simulink model "BasicQuadrotorControl"  (R2015a)
settings: Solver=FixedStepDiscrete  StartTime=0.0  StopTime=100000  RelTol=1e-3
model workspace (MAT data in the model file):
  clk_freq = Simulink.Parameter
  clk_freq.Value = 1000000
  clk_freq.DataType = 'uint32'
  cs_to_clk_edge = Simulink.Parameter
  cs_to_clk_edge.Value = 10
  cs_to_clk_edge.DataType = 'uint16'
  DATA_FORMAT = 12552
  init_cmd_ADXL = [11528 11528 11528 12552 12552]
  message_length = Simulink.Parameter
  message_length.Value = 16
  message_length.DataType = 'uint16'
  OUT_X_H = 45824
  OUT_X_L = 45568
  OUT_Y_H = 46336
  OUT_Y_L = 46080
  OUT_Z_H = 46848
  OUT_Z_L = 46592
  POWER_CTRL = 11528
  read_table_ADXL = [45568 45824 46080 46336 46592 46848 32768]
  stall_time = Simulink.Parameter
  stall_time.Value = 4
  stall_time.DataType = 'uint16'
  CTRL_REG1_L3G = 8399
  init_cmd_L3G = 8399
  OUT_X_H_L3G = 43264
  OUT_X_L_L3G = 43008
  OUT_Y_H_L3G = 43776
  OUT_Y_L_L3G = 43520
  OUT_Z_H_L3G = 44288
  OUT_Z_L_L3G = 44032
  read_table_L3G = [43008 43264 43520 43776 44032 44288 36608]
  WHO_AM_I_L3G = 36608
undefined symbols (not defined in the file): read_table
libraries: simulink x20, hdlsllib x2
settings Model: CovSFcnEnable=off  Creator=bsoheili  LastModifiedBy=dlwalter
settings DataIOCC: SaveOutput=off  SaveTime=off
settings OptimizationCC: BlockReduction=off  ConditionallyExecuteInputs=off  InlineParams=on  UseDivisionForNetSlopeComputation=UseDivisionForReciprocalsOfIntegersOnly  UseFloatMulNetSlope=on  InlineInvariantSignals=on  EnhancedBackFolding=on  EfficientFloat2IntCast=on  OptimizeModelRefInitCode=on  LifeSpan=1
settings DebuggingCC: AlgebraicLoopMsg=error  SolverPrmCheckMsg=warning  InheritedTsInSrcMsg=none  StrictBusMsg=ErrorOnBusTreatedAsVector  NonBusSignalsTreatedAsBus=error
settings HardwareCC: ProdHWDeviceType=ASIC/FPGA->ASIC/FPGA  ProdEqTarget=off
settings RTWCC: SystemTargetFile=ert.tlc  TemplateMakefile=ert_default_tmf  Description=Embedded Coder  GenerateReport=on  IncludeHyperlinkInReport=on  LaunchReport=on  GenerateTraceInfo=on  GenerateTraceReport=on  GenerateTraceReportSl=on  GenerateTraceReportSf=on  GenerateTraceReportEml=on  GenerateCodeMetricsReport=on
settings CodeAppCC: IgnoreCustomStorageClasses=off
settings ERTTargetCC: ParMdlRefBuildCompliant=on  CompOptLevelCompliant=on  ConcurrentExecutionCompliant=on  CombineSignalStateStructs=on  SuppressErrorStatus=on  ERTFirstTimeCompliant=on  SupportContinuousTime=off  SupportVariableSizeSignals=off  ModelStepFunctionPrototypeControlCompliant=on  CPPClassGenCompliant=on  ERTCustomFileTemplate=example_file_process.tlc

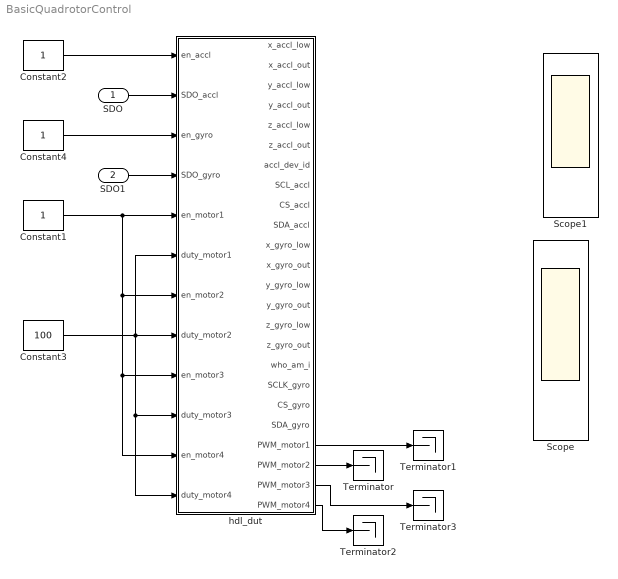
== system BasicQuadrotorControl ==
  SDO : Inport  OutDataTypeStr=boolean
  SDO1 : Inport  Port=2  OutDataTypeStr=boolean
  Constant1 : Constant  OutDataTypeStr=boolean  SampleTime=-1
  Constant2 : Constant  OutDataTypeStr=boolean  SampleTime=-1
  Constant3 : Constant  Value=100  OutDataTypeStr=uint8  SampleTime=-1
  Constant4 : Constant  OutDataTypeStr=boolean  SampleTime=-1
  Scope : Scope  NumInputPorts=4
      settings: TickLabels=on  TimeRange=2000  YMin=-5~-5~-5~-5  YMax=5~5~5~5
  Scope1 : Scope  NumInputPorts=4
      settings: TickLabels=on  TimeRange=2000  YMin=-5~-5~-5~-5  YMax=5~5~5~5  SaveName=ScopeData2
  Terminator{,1..3} (4 alike) : Terminator
  hdl_dut : Subsystem  TreatAsAtomicUnit=on
  wires:
  SDO/1 -> hdl_dut/2(SDO_accl)
  Constant3/1 -> hdl_dut/6(duty_motor1), hdl_dut/10(duty_motor3), hdl_dut/12(duty_motor4), hdl_dut/8(duty_motor2)
  Constant1/1 -> hdl_dut/5(en_motor1), hdl_dut/9(en_motor3), hdl_dut/11(en_motor4), hdl_dut/7(en_motor2)
  Constant2/1 -> hdl_dut/1(en_accl)
  Constant4/1 -> hdl_dut/3(en_gyro)
  SDO1/1 -> hdl_dut/4(SDO_gyro)
  hdl_dut/21(PWM_motor1) -> Terminator1/1
  hdl_dut/22(PWM_motor2) -> Terminator/1
  hdl_dut/23(PWM_motor3) -> Terminator3/1
  hdl_dut/24(PWM_motor4) -> Terminator2/1

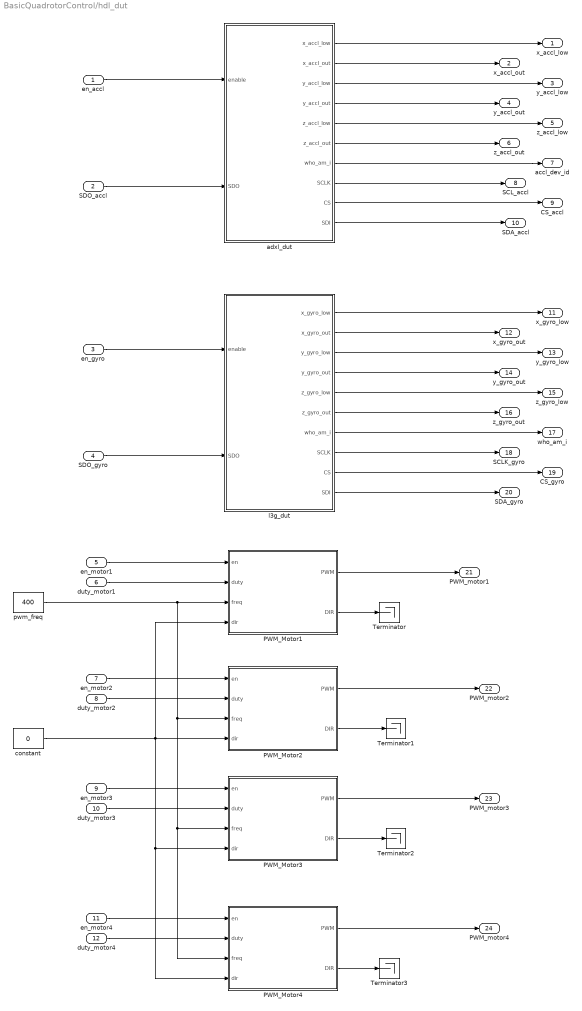
== system BasicQuadrotorControl/hdl_dut ==
  en_accl : Inport
  SDO_accl : Inport  Port=2
  en_gyro : Inport  Port=3
  SDO_gyro : Inport  Port=4
  en_motor1 : Inport  Port=5
  duty_motor1 : Inport  Port=6
  en_motor2 : Inport  Port=7
  duty_motor2 : Inport  Port=8
  en_motor3 : Inport  Port=9
  duty_motor3 : Inport  Port=10
  en_motor4 : Inport  Port=11
  duty_motor4 : Inport  Port=12
  PWM_Motor1 : Subsystem
  PWM_Motor2 : Subsystem
  PWM_Motor3 : Subsystem
  PWM_Motor4 : Subsystem
  Terminator{,1..3} (4 alike) : Terminator
  adxl_dut : Subsystem  TreatAsAtomicUnit=on  MinMaxOverflowLogging=MinMaxAndOverflow
  constant : Constant  Value=0  OutDataTypeStr=boolean  SampleTime=-1
  l3g_dut : Subsystem  TreatAsAtomicUnit=on  MinMaxOverflowLogging=MinMaxAndOverflow
  pwm_freq : Constant  Value=400  OutDataTypeStr=uint32  SampleTime=-1
  x_accl_low : Outport
  x_accl_out : Outport  Port=2
  y_accl_low : Outport  Port=3
  y_accl_out : Outport  Port=4
  z_accl_low : Outport  Port=5
  z_accl_out : Outport  Port=6
  accl_dev_id : Outport  Port=7
  SCL_accl : Outport  Port=8
  CS_accl : Outport  Port=9
  SDA_accl : Outport  Port=10
  x_gyro_low : Outport  Port=11
  x_gyro_out : Outport  Port=12
  y_gyro_low : Outport  Port=13
  y_gyro_out : Outport  Port=14
  z_gyro_low : Outport  Port=15
  z_gyro_out : Outport  Port=16
  who_am_i : Outport  Port=17
  SCLK_gyro : Outport  Port=18
  CS_gyro : Outport  Port=19
  SDA_gyro : Outport  Port=20
  PWM_motor1 : Outport  Port=21  OutDataTypeStr=boolean
  PWM_motor2 : Outport  Port=22  OutDataTypeStr=boolean
  PWM_motor3 : Outport  Port=23  OutDataTypeStr=boolean
  PWM_motor4 : Outport  Port=24  OutDataTypeStr=boolean
  wires:
  en_accl/1 -> adxl_dut/1(enable)
  SDO_accl/1 -> adxl_dut/2(SDO)
  adxl_dut/3(y_accl_low) -> y_accl_low/1
  adxl_dut/1(x_accl_low) -> x_accl_low/1
  pwm_freq/1 -> PWM_Motor4/3(freq), PWM_Motor3/3(freq), PWM_Motor2/3(freq), PWM_Motor1/3(freq)
  en_motor1/1 -> PWM_Motor1/1(en)
  duty_motor1/1 -> PWM_Motor1/2(duty)
  en_motor2/1 -> PWM_Motor2/1(en)
  duty_motor2/1 -> PWM_Motor2/2(duty)
  constant/1 -> PWM_Motor2/4(dir), PWM_Motor3/4(dir), PWM_Motor4/4(dir), PWM_Motor1/4(dir)
  PWM_Motor1/1(PWM) -> PWM_motor1/1
  PWM_Motor2/1(PWM) -> PWM_motor2/1
  PWM_Motor1/2(DIR) -> Terminator/1
  PWM_Motor2/2(DIR) -> Terminator1/1
  PWM_Motor3/2(DIR) -> Terminator2/1
  PWM_Motor4/2(DIR) -> Terminator3/1
  PWM_Motor3/1(PWM) -> PWM_motor3/1
  PWM_Motor4/1(PWM) -> PWM_motor4/1
  en_motor3/1 -> PWM_Motor3/1(en)
  duty_motor3/1 -> PWM_Motor3/2(duty)
  en_motor4/1 -> PWM_Motor4/1(en)
  duty_motor4/1 -> PWM_Motor4/2(duty)
  adxl_dut/10(SDI) -> SDA_accl/1
  adxl_dut/8(SCLK) -> SCL_accl/1
  adxl_dut/2(x_accl_out) -> x_accl_out/1
  adxl_dut/4(y_accl_out) -> y_accl_out/1
  adxl_dut/5(z_accl_low) -> z_accl_low/1
  adxl_dut/6(z_accl_out) -> z_accl_out/1
  adxl_dut/7(who_am_i) -> accl_dev_id/1
  en_gyro/1 -> l3g_dut/1(enable)
  SDO_gyro/1 -> l3g_dut/2(SDO)
  l3g_dut/10(SDI) -> SDA_gyro/1
  l3g_dut/8(SCLK) -> SCLK_gyro/1
  l3g_dut/1(x_gyro_low) -> x_gyro_low/1
  l3g_dut/2(x_gyro_out) -> x_gyro_out/1
  l3g_dut/3(y_gyro_low) -> y_gyro_low/1
  l3g_dut/4(y_gyro_out) -> y_gyro_out/1
  l3g_dut/5(z_gyro_low) -> z_gyro_low/1
  l3g_dut/6(z_gyro_out) -> z_gyro_out/1
  l3g_dut/7(who_am_i) -> who_am_i/1
  adxl_dut/9(CS) -> CS_accl/1
  l3g_dut/9(CS) -> CS_gyro/1

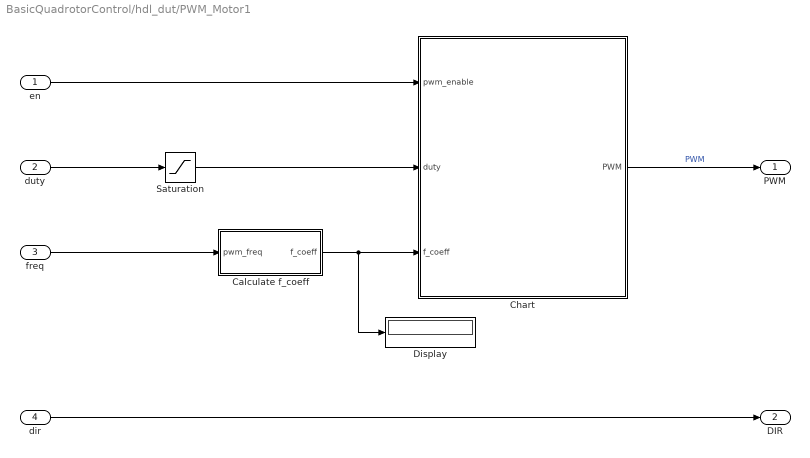
== system BasicQuadrotorControl/hdl_dut/PWM_Motor1 ==
  en : Inport  OutDataTypeStr=boolean  PortDimensions=1  SampleTime=[1,0]
  duty : Inport  Port=2  OutDataTypeStr=uint8  PortDimensions=1  SampleTime=[1,0]
  freq : Inport  Port=3  OutDataTypeStr=uint32  PortDimensions=1  SampleTime=[1,0]
  dir : Inport  Port=4  OutDataTypeStr=boolean  PortDimensions=1  SampleTime=[1,0]
  Calculate f_coeff : Subsystem  TreatAsAtomicUnit=on
  Chart : Stateflow chart  TreatAsAtomicUnit=on
  Display : Display
  Saturation : Saturate  UpperLimit=255  LowerLimit=0  OutDataTypeStr=fixdt(0,8,0)
  PWM : Outport  OutDataTypeStr=boolean  PortDimensions=1  SampleTime=[1,0]
  DIR : Outport  Port=2  PortDimensions=1  SampleTime=[1,0]
  wires:
  dir/1 -> DIR/1
  en/1 -> Chart/1(pwm_enable)
  duty/1 -> Saturation/1
  Saturation/1 -> Chart/2(duty)
  Chart/1(PWM) -> PWM/1  "PWM"
  freq/1 -> Calculate f_coeff/1(pwm_freq)
  Calculate f_coeff/1(f_coeff) -> Chart/3(f_coeff), Display/1

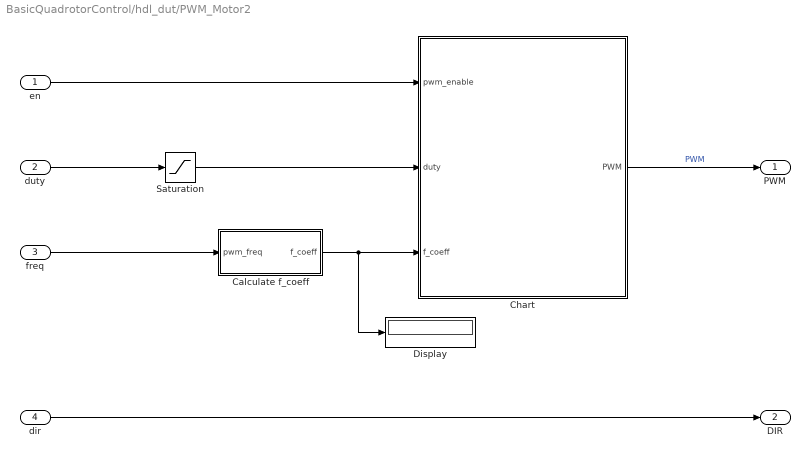
== system BasicQuadrotorControl/hdl_dut/PWM_Motor2 ==
  en : Inport  OutDataTypeStr=boolean  PortDimensions=1  SampleTime=[1,0]
  duty : Inport  Port=2  OutDataTypeStr=uint8  PortDimensions=1  SampleTime=[1,0]
  freq : Inport  Port=3  OutDataTypeStr=uint32  PortDimensions=1  SampleTime=[1,0]
  dir : Inport  Port=4  OutDataTypeStr=boolean  PortDimensions=1  SampleTime=[1,0]
  Calculate f_coeff : Subsystem  TreatAsAtomicUnit=on
  Chart : Stateflow chart  TreatAsAtomicUnit=on
  Display : Display
  Saturation : Saturate  UpperLimit=255  LowerLimit=0  OutDataTypeStr=fixdt(0,8,0)
  PWM : Outport  OutDataTypeStr=boolean  PortDimensions=1  SampleTime=[1,0]
  DIR : Outport  Port=2  PortDimensions=1  SampleTime=[1,0]
  wires:
  Calculate f_coeff/1(f_coeff) -> Display/1, Chart/3(f_coeff)
  freq/1 -> Calculate f_coeff/1(pwm_freq)
  Chart/1(PWM) -> PWM/1  "PWM"
  Saturation/1 -> Chart/2(duty)
  duty/1 -> Saturation/1
  en/1 -> Chart/1(pwm_enable)
  dir/1 -> DIR/1

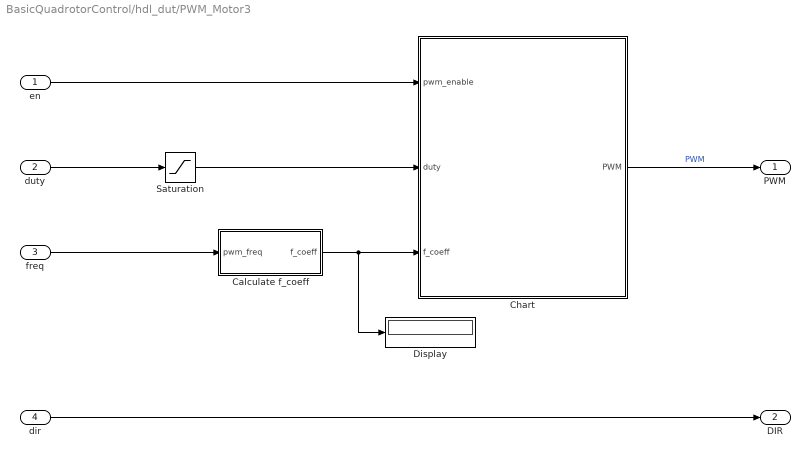
== system BasicQuadrotorControl/hdl_dut/PWM_Motor3 ==
  en : Inport  OutDataTypeStr=boolean  PortDimensions=1  SampleTime=[1,0]
  duty : Inport  Port=2  OutDataTypeStr=uint8  PortDimensions=1  SampleTime=[1,0]
  freq : Inport  Port=3  OutDataTypeStr=uint32  PortDimensions=1  SampleTime=[1,0]
  dir : Inport  Port=4  OutDataTypeStr=boolean  PortDimensions=1  SampleTime=[1,0]
  Calculate f_coeff : Subsystem  TreatAsAtomicUnit=on
  Chart : Stateflow chart  TreatAsAtomicUnit=on
  Display : Display
  Saturation : Saturate  UpperLimit=255  LowerLimit=0  OutDataTypeStr=fixdt(0,8,0)
  PWM : Outport  OutDataTypeStr=boolean  PortDimensions=1  SampleTime=[1,0]
  DIR : Outport  Port=2  PortDimensions=1  SampleTime=[1,0]
  wires:
  dir/1 -> DIR/1
  en/1 -> Chart/1(pwm_enable)
  duty/1 -> Saturation/1
  Saturation/1 -> Chart/2(duty)
  Chart/1(PWM) -> PWM/1  "PWM"
  freq/1 -> Calculate f_coeff/1(pwm_freq)
  Calculate f_coeff/1(f_coeff) -> Chart/3(f_coeff), Display/1

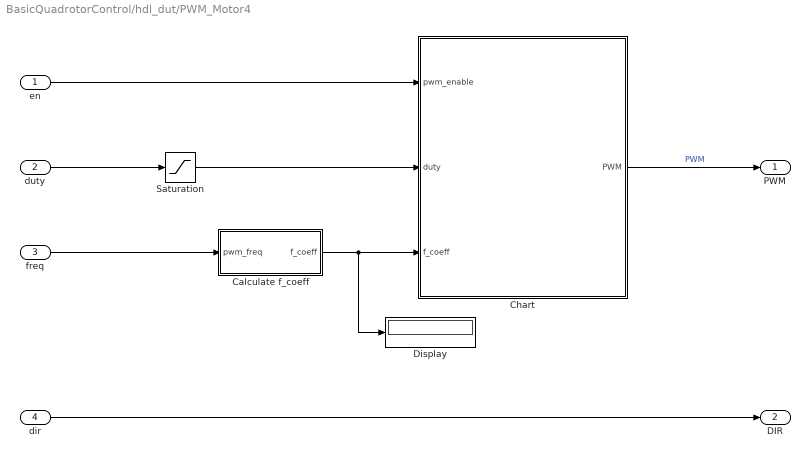
== system BasicQuadrotorControl/hdl_dut/PWM_Motor4 ==
  en : Inport  OutDataTypeStr=boolean  PortDimensions=1  SampleTime=[1,0]
  duty : Inport  Port=2  OutDataTypeStr=uint8  PortDimensions=1  SampleTime=[1,0]
  freq : Inport  Port=3  OutDataTypeStr=uint32  PortDimensions=1  SampleTime=[1,0]
  dir : Inport  Port=4  OutDataTypeStr=boolean  PortDimensions=1  SampleTime=[1,0]
  Calculate f_coeff : Subsystem  TreatAsAtomicUnit=on
  Chart : Stateflow chart  TreatAsAtomicUnit=on
  Display : Display
  Saturation : Saturate  UpperLimit=255  LowerLimit=0  OutDataTypeStr=fixdt(0,8,0)
  PWM : Outport  OutDataTypeStr=boolean  PortDimensions=1  SampleTime=[1,0]
  DIR : Outport  Port=2  PortDimensions=1  SampleTime=[1,0]
  wires:
  Calculate f_coeff/1(f_coeff) -> Display/1, Chart/3(f_coeff)
  freq/1 -> Calculate f_coeff/1(pwm_freq)
  Chart/1(PWM) -> PWM/1  "PWM"
  Saturation/1 -> Chart/2(duty)
  duty/1 -> Saturation/1
  en/1 -> Chart/1(pwm_enable)
  dir/1 -> DIR/1

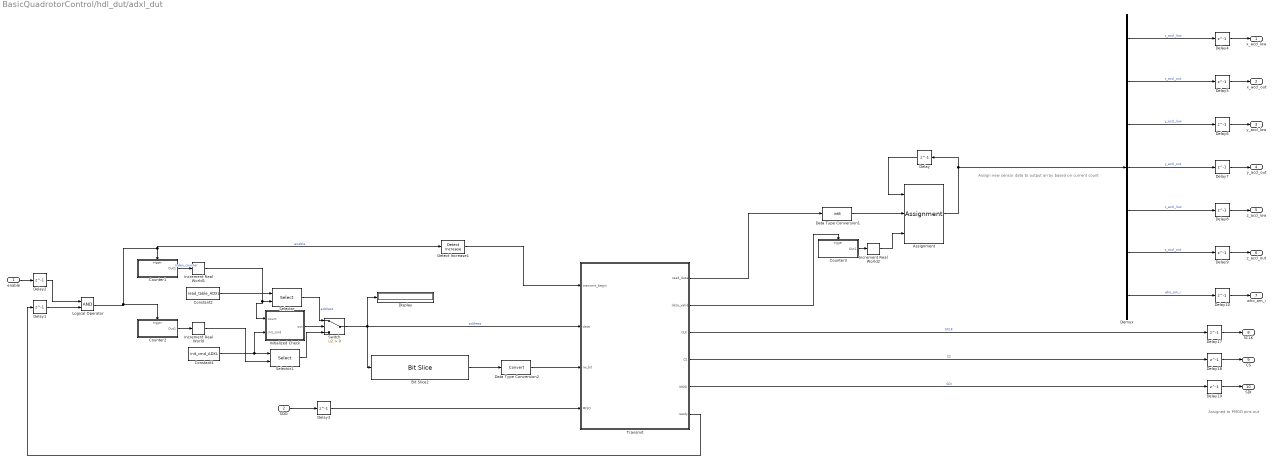
== system BasicQuadrotorControl/hdl_dut/adxl_dut ==
  note: Assign new sensor data to output array based on current count
  note: Assigned to PMOD pins out
  enable : Inport
  SDO : Inport  Port=2
  Assignment : Assignment  DiagnosticForDimensions=Warning  IndexOptions=Index vector (port)  OutputSizes=size(read_table,2)
  Bit Slice2 : hdlsllib/HDL Operations/Bit Slice  lidx=message_length-1  ridx=message_length-1
  Constant1 : Constant  Value=init_cmd_ADXL  OutDataTypeStr=uint16  SampleTime=1
  Constant2 : Constant  Value=read_table_ADXL  OutDataTypeStr=uint16  SampleTime=1
  Counter1 : Subsystem  TreatAsAtomicUnit=on
  Counter2 : Subsystem  TreatAsAtomicUnit=on
  Counter3 : Subsystem  TreatAsAtomicUnit=on
  Data Type Conversion1 : DataTypeConversion  OutDataTypeStr=int8  ConvertRealWorld=Stored Integer (SI)
  Data Type Conversion2 : DataTypeConversion
  Delay : Delay  DelayLength=1  InitialCondition=zeros(1,size(read_table_ADXL,2))  SampleTime=1
  Delay1 : Delay  DelayLength=1  InitialCondition=1
  Delay{4..10,17..19} (10 alike) : Delay  DelayLength=1  InitialCondition=0
  Delay2 : Delay  DelayLength=1  InitialCondition=1
  Delay3 : Delay  DelayLength=1  InitialCondition=1
  Demux : Demux  Outputs=7
  Detect Increase1 : simulink/Logic and Bit Operations/Detect Increase  vinit=0  InputProcessing=Inherited  OutDataTypeStr=boolean
  Display : Display
      settings: Format=binary (Stored Integer)
  Increment Real World : simulink/Additional Math & Discrete/Additional Math: Increment - Decrement/Increment Real World
  Increment Real World1 : simulink/Additional Math & Discrete/Additional Math: Increment - Decrement/Increment Real World
  Increment Real World2 : simulink/Additional Math & Discrete/Additional Math: Increment - Decrement/Increment Real World
  Initialized Check : MATLAB Function  TreatAsAtomicUnit=on
  Logical Operator : Logic  AllPortsSameDT=off  OutDataTypeStr=boolean
  Selector : Selector  InputPortWidth=size(read_table_ADXL,2)  IndexOptions=Index vector (port)  Indices=[1 3]
  Selector1 : Selector  InputPortWidth=size(init_cmd_ADXL,2)  IndexOptions=Index vector (port)  Indices=[1 3]
  Switch : Switch  Criteria=u2 > Threshold
  Transmit : Stateflow chart  TreatAsAtomicUnit=on
  x_accl_low : Outport
  x_accl_out : Outport  Port=2
  y_accl_low : Outport  Port=3
  y_accl_out : Outport  Port=4
  z_accl_low : Outport  Port=5
  z_accl_out : Outport  Port=6
  who_am_i : Outport  Port=7
  SCLK : Outport  Port=8
  CS : Outport  Port=9
  SDI : Outport  Port=10
  wires:
  Transmit/3(CLK) -> Delay17/1  "SCLK"
  Transmit/4(CS) -> Delay18/1  "CS"
  Transmit/5(MOSI) -> Delay19/1  "SDI"
  Assignment/1 -> Delay/1, Demux/1
  enable/1 -> Delay2/1
  Constant2/1 -> Selector/1
  Transmit/6(ready) -> Delay1/1
  SDO/1 -> Delay3/1
  Delay1/1 -> Logical Operator/2
  Counter1/1(Out1) -> Increment Real World1/1  "index_counter"
  Delay/1 -> Assignment/1
  Delay2/1 -> Logical Operator/1
  Delay4/1 -> x_accl_low/1
  Delay5/1 -> x_accl_out/1
  Delay6/1 -> y_accl_low/1
  Delay7/1 -> y_accl_out/1
  Delay8/1 -> z_accl_low/1
  Delay9/1 -> z_accl_out/1
  Delay10/1 -> who_am_i/1
  Delay17/1 -> SCLK/1
  Delay18/1 -> CS/1
  Delay19/1 -> SDI/1
  Detect Increase1/1 -> Transmit/1(transmit_begin)
  Logical Operator/1 -> Counter2/Trigger, Counter1/Trigger, Detect Increase1/1  "enable"
  Delay3/1 -> Transmit/4(MISO)
  Data Type Conversion2/1 -> Transmit/3(rw_bit)
  Switch/1 -> Display/1, Transmit/2(data), Bit Slice2/1  "address"
  Bit Slice2/1 -> Data Type Conversion2/1
  Demux/1 -> Delay4/1  "x_accl_low"
  Demux/2 -> Delay5/1  "x_accl_out"
  Demux/3 -> Delay6/1  "y_accl_low"
  Demux/4 -> Delay7/1  "y_accl_out"
  Demux/5 -> Delay8/1  "z_accl_low"
  Demux/6 -> Delay9/1  "z_accl_out"
  Demux/7 -> Delay10/1  "who_am_i"
  Transmit/1(read_data) -> Data Type Conversion1/1
  Data Type Conversion1/1 -> Assignment/2
  Counter3/1(Out1) -> Increment Real World2/1
  Transmit/2(data_valid) -> Counter3/Trigger
  Selector/1 -> Switch/1  "address"
  Selector1/1 -> Switch/3
  Constant1/1 -> Selector1/1, Initialized Check/2(init_cmd)
  Counter2/1(Out1) -> Increment Real World/1
  Increment Real World/1 -> Selector1/2
  Increment Real World1/1 -> Initialized Check/1(count), Selector/2
  Increment Real World2/1 -> Assignment/3
  Initialized Check/1(out) -> Switch/2

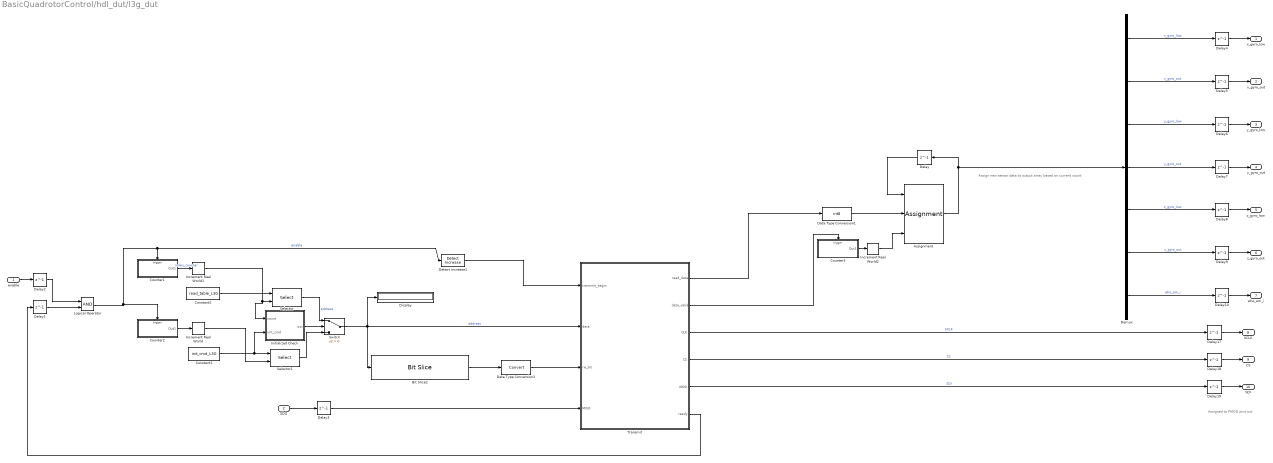
== system BasicQuadrotorControl/hdl_dut/l3g_dut ==
  note: Assign new sensor data to output array based on current count
  note: Assigned to PMOD pins out
  enable : Inport
  SDO : Inport  Port=2
  Assignment : Assignment  DiagnosticForDimensions=Warning  IndexOptions=Index vector (port)  OutputSizes=size(read_table,2)
  Bit Slice2 : hdlsllib/HDL Operations/Bit Slice  lidx=message_length-1  ridx=message_length-1
  Constant1 : Constant  Value=init_cmd_L3G  OutDataTypeStr=uint16  SampleTime=1
  Constant2 : Constant  Value=read_table_L3G  OutDataTypeStr=uint16  SampleTime=1
  Counter1 : Subsystem  TreatAsAtomicUnit=on
  Counter2 : Subsystem  TreatAsAtomicUnit=on
  Counter3 : Subsystem  TreatAsAtomicUnit=on
  Data Type Conversion1 : DataTypeConversion  OutDataTypeStr=int8  ConvertRealWorld=Stored Integer (SI)
  Data Type Conversion2 : DataTypeConversion
  Delay : Delay  DelayLength=1  InitialCondition=zeros(1,size(read_table_L3G,2))  SampleTime=1
  Delay1 : Delay  DelayLength=1  InitialCondition=1
  Delay{4..10,17..19} (10 alike) : Delay  DelayLength=1  InitialCondition=0
  Delay2 : Delay  DelayLength=1  InitialCondition=1
  Delay3 : Delay  DelayLength=1  InitialCondition=1
  Demux : Demux  Outputs=7
  Detect Increase1 : simulink/Logic and Bit Operations/Detect Increase  vinit=0  InputProcessing=Inherited  OutDataTypeStr=boolean
  Display : Display
      settings: Format=binary (Stored Integer)
  Increment Real World : simulink/Additional Math & Discrete/Additional Math: Increment - Decrement/Increment Real World
  Increment Real World1 : simulink/Additional Math & Discrete/Additional Math: Increment - Decrement/Increment Real World
  Increment Real World2 : simulink/Additional Math & Discrete/Additional Math: Increment - Decrement/Increment Real World
  Initialized Check : MATLAB Function  TreatAsAtomicUnit=on
  Logical Operator : Logic  AllPortsSameDT=off  OutDataTypeStr=boolean
  Selector : Selector  InputPortWidth=size(read_table_L3G,2)  IndexOptions=Index vector (port)  Indices=[1 3]
  Selector1 : Selector  InputPortWidth=size(init_cmd_L3G,2)  IndexOptions=Index vector (port)  Indices=[1 3]
  Switch : Switch  Criteria=u2 > Threshold
  Transmit : Stateflow chart  TreatAsAtomicUnit=on
  x_gyro_low : Outport
  x_gyro_out : Outport  Port=2
  y_gyro_low : Outport  Port=3
  y_gyro_out : Outport  Port=4
  z_gyro_low : Outport  Port=5
  z_gyro_out : Outport  Port=6
  who_am_i : Outport  Port=7
  SCLK : Outport  Port=8
  CS : Outport  Port=9
  SDI : Outport  Port=10
  wires:
  Transmit/3(CLK) -> Delay17/1  "SCLK"
  Transmit/4(CS) -> Delay18/1  "CS"
  Transmit/5(MOSI) -> Delay19/1  "SDI"
  Assignment/1 -> Delay/1, Demux/1
  enable/1 -> Delay2/1
  Constant2/1 -> Selector/1
  Transmit/6(ready) -> Delay1/1
  SDO/1 -> Delay3/1
  Delay1/1 -> Logical Operator/2
  Counter1/1(Out1) -> Increment Real World1/1  "index_counter"
  Delay/1 -> Assignment/1
  Delay2/1 -> Logical Operator/1
  Delay4/1 -> x_gyro_low/1
  Delay5/1 -> x_gyro_out/1
  Delay6/1 -> y_gyro_low/1
  Delay7/1 -> y_gyro_out/1
  Delay8/1 -> z_gyro_low/1
  Delay9/1 -> z_gyro_out/1
  Delay10/1 -> who_am_i/1
  Delay17/1 -> SCLK/1
  Delay18/1 -> CS/1
  Delay19/1 -> SDI/1
  Detect Increase1/1 -> Transmit/1(transmit_begin)
  Logical Operator/1 -> Counter2/Trigger, Counter1/Trigger, Detect Increase1/1  "enable"
  Delay3/1 -> Transmit/4(MISO)
  Data Type Conversion2/1 -> Transmit/3(rw_bit)
  Switch/1 -> Display/1, Transmit/2(data), Bit Slice2/1  "address"
  Bit Slice2/1 -> Data Type Conversion2/1
  Demux/1 -> Delay4/1  "x_gyro_low"
  Demux/2 -> Delay5/1  "x_gyro_out"
  Demux/3 -> Delay6/1  "y_gyro_low"
  Demux/4 -> Delay7/1  "y_gyro_out"
  Demux/5 -> Delay8/1  "z_gyro_low"
  Demux/6 -> Delay9/1  "z_gyro_out"
  Demux/7 -> Delay10/1  "who_am_i"
  Transmit/1(read_data) -> Data Type Conversion1/1
  Data Type Conversion1/1 -> Assignment/2
  Counter3/1(Out1) -> Increment Real World2/1
  Transmit/2(data_valid) -> Counter3/Trigger
  Selector/1 -> Switch/1  "address"
  Selector1/1 -> Switch/3
  Constant1/1 -> Selector1/1, Initialized Check/2(init_cmd)
  Counter2/1(Out1) -> Increment Real World/1
  Increment Real World/1 -> Selector1/2
  Increment Real World1/1 -> Initialized Check/1(count), Selector/2
  Increment Real World2/1 -> Assignment/3
  Initialized Check/1(out) -> Switch/2

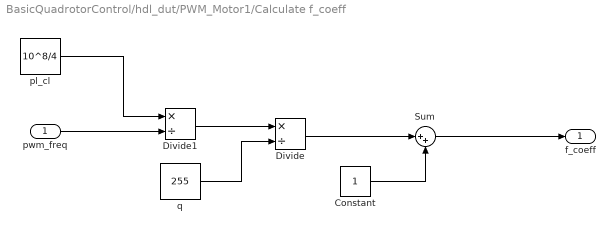
== system BasicQuadrotorControl/hdl_dut/PWM_Motor1/Calculate f_coeff ==
  pwm_freq : Inport
  Constant : Constant  OutDataTypeStr=uint32
  Divide : Product  Inputs=*/  SaturateOnIntegerOverflow=on  RndMeth=Zero
  Divide1 : Product  Inputs=*/  SaturateOnIntegerOverflow=on  RndMeth=Zero
  Sum : Sum  Inputs=|++  AccumDataTypeStr=uint32  RndMeth=Zero
  pl_cl : Constant  Value=10^8/4  OutDataTypeStr=uint32
  q : Constant  Value=255  OutDataTypeStr=Inherit: Inherit via back propagation
  f_coeff : Outport  OutDataTypeStr=uint32
  wires:
  Constant/1 -> Sum/2
  Sum/1 -> f_coeff/1
  Divide/1 -> Sum/1
  pl_cl/1 -> Divide1/1
  pwm_freq/1 -> Divide1/2
  Divide1/1 -> Divide/1
  q/1 -> Divide/2

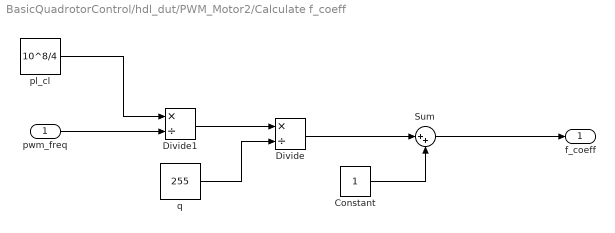
== system BasicQuadrotorControl/hdl_dut/PWM_Motor2/Calculate f_coeff ==
  pwm_freq : Inport
  Constant : Constant  OutDataTypeStr=uint32
  Divide : Product  Inputs=*/  SaturateOnIntegerOverflow=on  RndMeth=Zero
  Divide1 : Product  Inputs=*/  SaturateOnIntegerOverflow=on  RndMeth=Zero
  Sum : Sum  Inputs=|++  AccumDataTypeStr=uint32  RndMeth=Zero
  pl_cl : Constant  Value=10^8/4  OutDataTypeStr=uint32
  q : Constant  Value=255  OutDataTypeStr=Inherit: Inherit via back propagation
  f_coeff : Outport  OutDataTypeStr=uint32
  wires:
  q/1 -> Divide/2
  Divide1/1 -> Divide/1
  pwm_freq/1 -> Divide1/2
  pl_cl/1 -> Divide1/1
  Divide/1 -> Sum/1
  Sum/1 -> f_coeff/1
  Constant/1 -> Sum/2

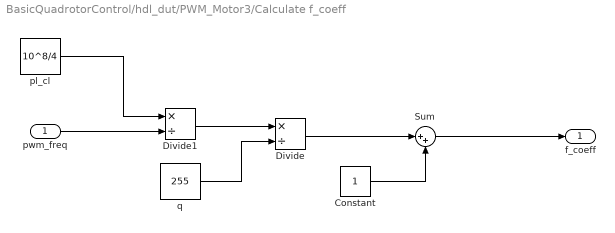
== system BasicQuadrotorControl/hdl_dut/PWM_Motor3/Calculate f_coeff ==
  pwm_freq : Inport
  Constant : Constant  OutDataTypeStr=uint32
  Divide : Product  Inputs=*/  SaturateOnIntegerOverflow=on  RndMeth=Zero
  Divide1 : Product  Inputs=*/  SaturateOnIntegerOverflow=on  RndMeth=Zero
  Sum : Sum  Inputs=|++  AccumDataTypeStr=uint32  RndMeth=Zero
  pl_cl : Constant  Value=10^8/4  OutDataTypeStr=uint32
  q : Constant  Value=255  OutDataTypeStr=Inherit: Inherit via back propagation
  f_coeff : Outport  OutDataTypeStr=uint32
  wires:
  Constant/1 -> Sum/2
  Sum/1 -> f_coeff/1
  Divide/1 -> Sum/1
  pl_cl/1 -> Divide1/1
  pwm_freq/1 -> Divide1/2
  Divide1/1 -> Divide/1
  q/1 -> Divide/2

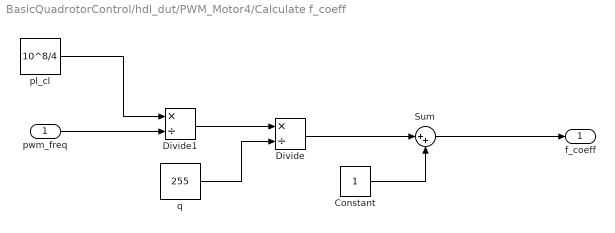
== system BasicQuadrotorControl/hdl_dut/PWM_Motor4/Calculate f_coeff ==
  pwm_freq : Inport
  Constant : Constant  OutDataTypeStr=uint32
  Divide : Product  Inputs=*/  SaturateOnIntegerOverflow=on  RndMeth=Zero
  Divide1 : Product  Inputs=*/  SaturateOnIntegerOverflow=on  RndMeth=Zero
  Sum : Sum  Inputs=|++  AccumDataTypeStr=uint32  RndMeth=Zero
  pl_cl : Constant  Value=10^8/4  OutDataTypeStr=uint32
  q : Constant  Value=255  OutDataTypeStr=Inherit: Inherit via back propagation
  f_coeff : Outport  OutDataTypeStr=uint32
  wires:
  q/1 -> Divide/2
  Divide1/1 -> Divide/1
  pwm_freq/1 -> Divide1/2
  pl_cl/1 -> Divide1/1
  Divide/1 -> Sum/1
  Sum/1 -> f_coeff/1
  Constant/1 -> Sum/2

== system BasicQuadrotorControl/hdl_dut/adxl_dut/Counter1 ==
  Trigger : TriggerPort  PortDimensions=1
  Delay : Delay  DelayLength=1  InitialCondition=1
  Increment Real World : simulink/Additional Math & Discrete/Additional Math: Increment - Decrement/Increment Real World
  Wrap To Zero : simulink/Discontinuities/Wrap To Zero  DisableCoverage=on  Threshold=size(read_table_ADXL,2)-1
  Out1 : Outport  OutDataTypeStr=int16  InitialOutput=0
  wires:
  Delay/1 -> Wrap To Zero/1
  Increment Real World/1 -> Delay/1
  Wrap To Zero/1 -> Out1/1, Increment Real World/1

== system BasicQuadrotorControl/hdl_dut/adxl_dut/Counter2 ==
  Trigger : TriggerPort  PortDimensions=1
  Delay : Delay  DelayLength=1  InitialCondition=1
  Increment Real World : simulink/Additional Math & Discrete/Additional Math: Increment - Decrement/Increment Real World
  Wrap To Zero : simulink/Discontinuities/Wrap To Zero  DisableCoverage=on  Threshold=size(init_cmd_ADXL,2)-1
  Out1 : Outport  OutDataTypeStr=int16  InitialOutput=0
  wires:
  Wrap To Zero/1 -> Increment Real World/1, Out1/1
  Increment Real World/1 -> Delay/1
  Delay/1 -> Wrap To Zero/1

== system BasicQuadrotorControl/hdl_dut/adxl_dut/Counter3 ==
  Trigger : TriggerPort  PortDimensions=1
  Delay : Delay  DelayLength=1  InitialCondition=0
  Increment Real World : simulink/Additional Math & Discrete/Additional Math: Increment - Decrement/Increment Real World
  Wrap To Zero : simulink/Discontinuities/Wrap To Zero  DisableCoverage=on  Threshold=size(read_table_ADXL,2)-1
  Out1 : Outport  OutDataTypeStr=int16  InitialOutput=0
  wires:
  Wrap To Zero/1 -> Increment Real World/1, Out1/1
  Increment Real World/1 -> Delay/1
  Delay/1 -> Wrap To Zero/1

== system BasicQuadrotorControl/hdl_dut/l3g_dut/Counter1 ==
  Trigger : TriggerPort  PortDimensions=1
  Delay : Delay  DelayLength=1  InitialCondition=1
  Increment Real World : simulink/Additional Math & Discrete/Additional Math: Increment - Decrement/Increment Real World
  Wrap To Zero : simulink/Discontinuities/Wrap To Zero  DisableCoverage=on  Threshold=size(read_table_L3G,2)-1
  Out1 : Outport  OutDataTypeStr=int16  InitialOutput=0
  wires:
  Delay/1 -> Wrap To Zero/1
  Increment Real World/1 -> Delay/1
  Wrap To Zero/1 -> Out1/1, Increment Real World/1

== system BasicQuadrotorControl/hdl_dut/l3g_dut/Counter2 ==
  Trigger : TriggerPort  PortDimensions=1
  Delay : Delay  DelayLength=1  InitialCondition=1
  Increment Real World : simulink/Additional Math & Discrete/Additional Math: Increment - Decrement/Increment Real World
  Wrap To Zero : simulink/Discontinuities/Wrap To Zero  DisableCoverage=on  Threshold=size(init_cmd_L3G,2)-1
  Out1 : Outport  OutDataTypeStr=int16  InitialOutput=0
  wires:
  Wrap To Zero/1 -> Increment Real World/1, Out1/1
  Increment Real World/1 -> Delay/1
  Delay/1 -> Wrap To Zero/1

== system BasicQuadrotorControl/hdl_dut/l3g_dut/Counter3 ==
  Trigger : TriggerPort  PortDimensions=1
  Delay : Delay  DelayLength=1  InitialCondition=0
  Increment Real World : simulink/Additional Math & Discrete/Additional Math: Increment - Decrement/Increment Real World
  Wrap To Zero : simulink/Discontinuities/Wrap To Zero  DisableCoverage=on  Threshold=size(read_table_L3G,2)-1
  Out1 : Outport  OutDataTypeStr=int16  InitialOutput=0
  wires:
  Wrap To Zero/1 -> Increment Real World/1, Out1/1
  Increment Real World/1 -> Delay/1
  Delay/1 -> Wrap To Zero/1

== stateflow chart BasicQuadrotorControl/hdl_dut/adxl_dut/Transmit ==
  settings: executeAtInitialization=1
  state IDLE
  state BEGIN
  state CHIPSELECT
  state WRITE
    state CLOCK_BEGIN
    state CLOCK_HIGH
    state CLOCK_LOW
    state CLOCK_END
    (default) -> CLOCK_BEGIN
    CLOCK_BEGIN -> CLOCK_LOW : {CLK = false;
        | bit_count = 0;
        | MOSI = sdi_gen(data,1);}
    CLOCK_LOW -> CLOCK_HIGH [order 1] : [count == clk_wait]
        | {CLK = 1; count = 0;bit_count ++;}
    CLOCK_HIGH -> CLOCK_HIGH [order 3] : {count++;}
    CLOCK_LOW -> CLOCK_LOW [order 2] : {count++;}
    CLOCK_HIGH -> CLOCK_LOW [order 1] : [count == clk_wait]
        | {CLK = 0; count = 0;
        | MOSI = sdi_gen(data, bit_count+1);}
    CLOCK_HIGH -> CLOCK_END [order 2] : [bit_count == message_length]
        | {count = 0; transmit_flag = 0; MOSI = 0; data_valid = 1;}
  state READ
    state CLOCK_BEGIN1
    state CLOCK_HIGH1
    state CLOCK_LOW1
    state CLOCK_LOW3
    state CLOCK_HIGH3
    state DATA_VALID1
    state CLK_END1
    (default) -> CLOCK_BEGIN1
    CLOCK_BEGIN1 -> CLOCK_LOW1 : {CLK = false;
        | bit_count = 0;
        | MOSI = sdi_gen(data, 1);}
    CLOCK_LOW1 -> CLOCK_HIGH1 [order 1] : [count == clk_wait]
        | {CLK = 1; count = 0;bit_count ++;}
    CLOCK_HIGH1 -> CLOCK_HIGH1 [order 2] : {count++;}
    CLOCK_LOW1 -> CLOCK_LOW1 [order 3] : {count++;}
    CLOCK_HIGH1 -> CLOCK_LOW1 [order 1] : [count == clk_wait]
        | {CLK = 0; count = 0;
        | MOSI = sdi_gen(data, bit_count+1);}
    CLOCK_LOW1 -> CLOCK_LOW3 [order 2] : [bit_count == message_length/2]
        | {count = 0; MOSI = 0; CLK = false;
        | read_temp = 0;}
    CLOCK_LOW3 -> CLOCK_HIGH3 [order 1] : [count == clk_wait]
        | {CLK = 1; count = 0;bit_count ++;
        | read_bit = int16(MISO);
        | read_temp = read_temp<<1;
        | read_temp = read_temp|read_bit;}
    CLOCK_HIGH3 -> CLOCK_HIGH3 [order 3] : {count++;}
    CLOCK_LOW3 -> CLOCK_LOW3 [order 2] : {count++;}
    CLOCK_HIGH3 -> CLOCK_LOW3 [order 1] : [count == clk_wait]
        | {CLK = 0; count = 0;}
    CLOCK_HIGH3 -> DATA_VALID1 [order 2] : [bit_count == message_length]
        | {count = 0; MOSI = 0; data_valid = 1;
        | read_data = read_temp;}
    DATA_VALID1 -> CLK_END1 : {transmit_flag = 0;}
  state END_TRANS
  state STALL
  (default) -> IDLE
  STALL -> IDLE [order 1] : [count == stall_wait]
      | {ready = 1;}
  IDLE -> BEGIN : [transmit_begin == 1]
      | {ready = 0;transmit_flag = 1;count = 0;CS = 1; CLK = 1;}
  BEGIN -> CHIPSELECT : {CS = 0;}
  CHIPSELECT -> CHIPSELECT [order 2] : {count++;}
  CHIPSELECT -> (junction 228) [order 1] : [count == cs_wait]{count = 0;}
  (junction 228) -> READ [order 1] : [rw_bit == READ_BIT]
  (junction 228) -> WRITE [order 2] : [rw_bit == WRITE_BIT]
  WRITE -> END_TRANS : [transmit_flag == 0]
      | {data_valid = 0;}
  READ -> END_TRANS : [transmit_flag == 0]
      | {data_valid = 0;}
  END_TRANS -> END_TRANS [order 2] : {count++;}
  END_TRANS -> STALL [order 1] : [count == cs_wait]{count = 0; CS = 1;}
  STALL -> STALL [order 2] : {count++;}
  data: word function_input fixdt(0,16,0); cnt function_input fixdt(0,5,0); ser_data function_output boolean; read_data output uint8; data_valid output boolean =0; CLK output boolean =true; CS output boolean =true; MOSI output boolean; clk_wait local fixdt(0,16,0) =floor(12.5e6/clk_freq); stall_wait local fixdt(0,16,0) =ceil(stall_time/.04); cs_wait local fixdt(0,16,0) =ceil(cs_to_clk_edge/40); count local fixdt(0,16,0); bit_count local fixdt(0,16,0); transmit_flag local boolean; read_bit local uint16; read_temp local uint16; transmit_begin input boolean; data input fixdt(0,message_length,0); rw_bit input boolean; MISO input boolean; clk_freq constant fixdt(0,32,0) =1e6; stall_time constant fixdt(0,16,0) =4; cs_to_clk_edge constant fixdt(0,32,0) =10; message_length constant fixdt(0,16,0) =16; ready output boolean =1; READ_BIT constant boolean =1; WRITE_BIT constant boolean =0
  function ser_data = sdi_gen(word,cnt):
    | function ser_data = sdi_gen(word,cnt)
    | 
    | 
    | persistent ser_data_int;
    | if isempty(ser_data_int)
    |     ser_data_int = false;
    | end
    | 
    | 
    | if cnt == fi(1,0,5,0)
    |     ser_data_int = logical(bitget(word, 16));
    | elseif cnt == fi(2,0,5,0)
    |     ser_data_int = logical(bitget(word, 15));
    | elseif cnt == fi(3,0,5,0)
    |     ser_data_int = logical(bitget(word, 14));
    | elseif cnt == fi(4,0,5,0)
    |     ser_data_int = logical(bitget(word, 13));
    | elseif cnt == fi(5,0,5,0)
    |     ser_data_int = logical(bitget(word, 12));
    | elseif cnt == fi(6,0,5,0)
    |     ser_data_int = logical(bitget(word, 11));
    | elseif cnt == fi(7,0,5,0)
    |     ser_data_int = logical(bitget(word, 10));
    | elseif cnt == fi(8,0,5,0)
    |     ser_data_int = logical(bitget(word, 9));
    | elseif cnt == fi(9,0,5,0)
    |     ser_data_int = logical(bitget(word, 8));
    | elseif cnt == fi(10,0,5,0)
    |     ser_data_int = logical(bitget(word, 7));
    | elseif cnt == fi(11,0,5,0)
    |     ser_data_int = logical(bitget(word, 6));
    | elseif cnt == fi(12,0,5,0)
    |     ser_data_int = logical(bitget(word, 5));
    | elseif cnt == fi(13,0,5,0)
    |     ser_data_int = logical(bitget(word, 4));
    | elseif cnt == fi(14,0,5,0)
    |     ser_data_int = logical(bitget(word, 3));
    | elseif cnt == fi(15,0,5,0)
    |     ser_data_int = logical(bitget(word, 2));
    | elseif cnt == fi(16,0,5,0)
    |     ser_data_int = logical(bitget(word, 1));    
    | else
    |     ser_data_int = true;
    | end
    | 
    | ser_data = ser_data_int;

== matlab function BasicQuadrotorControl/hdl_dut/adxl_dut/Initialized Check ==
  data: out output; count input; init_cmd input
function out = fcn(count, init_cmd)


persistent init_complete;
if isempty(init_complete)
    if count == fi(size(init_cmd,1)+1,0,16,0)  % set true after initialization is sent 
        out = false;
        init_complete = true;
    else
        out = false;
    end
else
        out = true;
    
end

== matlab function BasicQuadrotorControl/hdl_dut/l3g_dut/Initialized Check ==
  data: out output; count input; init_cmd input
function out = fcn(count, init_cmd)


persistent init_complete;
if isempty(init_complete)
    if count == fi(size(init_cmd,1)+1,0,16,0)  % set true after initialization is sent 
        out = false;
        init_complete = true;
    else
        out = false;
    end
else
        out = true;
    
end

== stateflow chart BasicQuadrotorControl/hdl_dut/PWM_Motor1/Chart ==
  settings: executeAtInitialization=1
  state S1
  note: The multiple of 40 for f_coeff raises the counts to 10,200 for one PWM wave, resulting in a frequency of 9804 Hz
      | Max PWM Frequency for the Cytron is 10 KHz
  state LOW
  state HIGH
  state S2
  (default) -> S1
  S2 -> S1
  S1 -> LOW : [pwm_enable == 1]{count = uint16(0); PWM = false;}
  LOW -> LOW [order 2] : {count = count + 1;}
  HIGH -> HIGH [order 3] : {count = count + 1;}
  LOW -> HIGH [order 1] : [count >= uint32(255-duty)*f_coeff && duty > 0]{PWM = true;}
  HIGH -> LOW [order 1] : [count >= uint32(255)*f_coeff && duty < 255]
      | {PWM = false; count = uint16(0);}
  LOW -> S2 [order 3] : [pwm_enable == 0]{PWM=false}
  HIGH -> S2 [order 2] : [pwm_enable == 0]{PWM = false;}
  data: PWM output boolean [0..1]; pwm_enable input [0..1]; count local; duty input; f_coeff input

== stateflow chart BasicQuadrotorControl/hdl_dut/PWM_Motor2/Chart ==
  settings: executeAtInitialization=1
  state S1
  note: The multiple of 40 for f_coeff raises the counts to 10,200 for one PWM wave, resulting in a frequency of 9804 Hz
      | Max PWM Frequency for the Cytron is 10 KHz
  state LOW
  state HIGH
  state S2
  (default) -> S1
  S2 -> S1
  S1 -> LOW : [pwm_enable == 1]{count = uint16(0); PWM = false;}
  LOW -> LOW [order 2] : {count = count + 1;}
  HIGH -> HIGH [order 3] : {count = count + 1;}
  LOW -> HIGH [order 1] : [count >= uint32(255-duty)*f_coeff && duty > 0]{PWM = true;}
  HIGH -> LOW [order 1] : [count >= uint32(255)*f_coeff && duty < 255]
      | {PWM = false; count = uint16(0);}
  LOW -> S2 [order 3] : [pwm_enable == 0]{PWM=false}
  HIGH -> S2 [order 2] : [pwm_enable == 0]{PWM = false;}
  data: PWM output boolean [0..1]; pwm_enable input [0..1]; count local; duty input; f_coeff input

== stateflow chart BasicQuadrotorControl/hdl_dut/PWM_Motor3/Chart ==
  settings: executeAtInitialization=1
  state S1
  note: The multiple of 40 for f_coeff raises the counts to 10,200 for one PWM wave, resulting in a frequency of 9804 Hz
      | Max PWM Frequency for the Cytron is 10 KHz
  state LOW
  state HIGH
  state S2
  (default) -> S1
  S2 -> S1
  S1 -> LOW : [pwm_enable == 1]{count = uint16(0); PWM = false;}
  LOW -> LOW [order 2] : {count = count + 1;}
  HIGH -> HIGH [order 3] : {count = count + 1;}
  LOW -> HIGH [order 1] : [count >= uint32(255-duty)*f_coeff && duty > 0]{PWM = true;}
  HIGH -> LOW [order 1] : [count >= uint32(255)*f_coeff && duty < 255]
      | {PWM = false; count = uint16(0);}
  LOW -> S2 [order 3] : [pwm_enable == 0]{PWM=false}
  HIGH -> S2 [order 2] : [pwm_enable == 0]{PWM = false;}
  data: PWM output boolean [0..1]; pwm_enable input [0..1]; count local; duty input; f_coeff input

== stateflow chart BasicQuadrotorControl/hdl_dut/PWM_Motor4/Chart ==
  settings: executeAtInitialization=1
  state S1
  note: The multiple of 40 for f_coeff raises the counts to 10,200 for one PWM wave, resulting in a frequency of 9804 Hz
      | Max PWM Frequency for the Cytron is 10 KHz
  state LOW
  state HIGH
  state S2
  (default) -> S1
  S2 -> S1
  S1 -> LOW : [pwm_enable == 1]{count = uint16(0); PWM = false;}
  LOW -> LOW [order 2] : {count = count + 1;}
  HIGH -> HIGH [order 3] : {count = count + 1;}
  LOW -> HIGH [order 1] : [count >= uint32(255-duty)*f_coeff && duty > 0]{PWM = true;}
  HIGH -> LOW [order 1] : [count >= uint32(255)*f_coeff && duty < 255]
      | {PWM = false; count = uint16(0);}
  LOW -> S2 [order 3] : [pwm_enable == 0]{PWM=false}
  HIGH -> S2 [order 2] : [pwm_enable == 0]{PWM = false;}
  data: PWM output boolean [0..1]; pwm_enable input [0..1]; count local; duty input; f_coeff input

== stateflow chart BasicQuadrotorControl/hdl_dut/l3g_dut/Transmit ==
  settings: executeAtInitialization=1
  state IDLE
  state BEGIN
  state CHIPSELECT
  state WRITE
    state CLOCK_BEGIN
    state CLOCK_HIGH
    state CLOCK_LOW
    state CLOCK_END
    (default) -> CLOCK_BEGIN
    CLOCK_BEGIN -> CLOCK_LOW : {CLK = false;
        | bit_count = 0;
        | MOSI = sdi_gen(data,1);}
    CLOCK_LOW -> CLOCK_HIGH [order 1] : [count == clk_wait]
        | {CLK = 1; count = 0;bit_count ++;}
    CLOCK_HIGH -> CLOCK_HIGH [order 3] : {count++;}
    CLOCK_LOW -> CLOCK_LOW [order 2] : {count++;}
    CLOCK_HIGH -> CLOCK_LOW [order 1] : [count == clk_wait]
        | {CLK = 0; count = 0;
        | MOSI = sdi_gen(data, bit_count+1);}
    CLOCK_HIGH -> CLOCK_END [order 2] : [bit_count == message_length]
        | {count = 0; transmit_flag = 0; MOSI = 0; data_valid = 1;}
  state READ
    state CLOCK_BEGIN1
    state CLOCK_HIGH1
    state CLOCK_LOW1
    state CLOCK_LOW3
    state CLOCK_HIGH3
    state DATA_VALID1
    state CLK_END1
    (default) -> CLOCK_BEGIN1
    CLOCK_BEGIN1 -> CLOCK_LOW1 : {CLK = false;
        | bit_count = 0;
        | MOSI = sdi_gen(data, 1);}
    CLOCK_LOW1 -> CLOCK_HIGH1 [order 1] : [count == clk_wait]
        | {CLK = 1; count = 0;bit_count ++;}
    CLOCK_HIGH1 -> CLOCK_HIGH1 [order 2] : {count++;}
    CLOCK_LOW1 -> CLOCK_LOW1 [order 3] : {count++;}
    CLOCK_HIGH1 -> CLOCK_LOW1 [order 1] : [count == clk_wait]
        | {CLK = 0; count = 0;
        | MOSI = sdi_gen(data, bit_count+1);}
    CLOCK_LOW1 -> CLOCK_LOW3 [order 2] : [bit_count == message_length/2]
        | {count = 0; MOSI = 0; CLK = false;
        | read_temp = 0;}
    CLOCK_LOW3 -> CLOCK_HIGH3 [order 1] : [count == clk_wait]
        | {CLK = 1; count = 0;bit_count ++;
        | read_bit = int16(MISO);
        | read_temp = read_temp<<1;
        | read_temp = read_temp|read_bit;}
    CLOCK_HIGH3 -> CLOCK_HIGH3 [order 3] : {count++;}
    CLOCK_LOW3 -> CLOCK_LOW3 [order 2] : {count++;}
    CLOCK_HIGH3 -> CLOCK_LOW3 [order 1] : [count == clk_wait]
        | {CLK = 0; count = 0;}
    CLOCK_HIGH3 -> DATA_VALID1 [order 2] : [bit_count == message_length]
        | {count = 0; MOSI = 0; data_valid = 1;
        | read_data = read_temp; }
    DATA_VALID1 -> CLK_END1 : {transmit_flag = 0;}
  state END_TRANS
  state STALL
  (default) -> IDLE
  STALL -> IDLE [order 1] : [count == stall_wait]
      | {ready = 1;}
  IDLE -> BEGIN : [transmit_begin == 1]
      | {ready = 0;transmit_flag = 1;count = 0;CS = 1; CLK = 1;}
  BEGIN -> CHIPSELECT : {CS = 0;}
  CHIPSELECT -> CHIPSELECT [order 2] : {count++;}
  CHIPSELECT -> (junction 228) [order 1] : [count == cs_wait]{count = 0;}
  (junction 228) -> READ [order 1] : [rw_bit == READ_BIT]
  (junction 228) -> WRITE [order 2] : [rw_bit == WRITE_BIT]
  WRITE -> END_TRANS : [transmit_flag == 0]
      | {data_valid = 0;}
  READ -> END_TRANS : [transmit_flag == 0]
      | {data_valid = 0;}
  END_TRANS -> END_TRANS [order 2] : {count++;}
  END_TRANS -> STALL [order 1] : [count == cs_wait]{count = 0; CS = 1;}
  STALL -> STALL [order 2] : {count++;}
  data: word function_input fixdt(0,16,0); cnt function_input fixdt(0,5,0); ser_data function_output boolean; read_data output uint8; data_valid output boolean =0; CLK output boolean =true; CS output boolean =true; MOSI output boolean; clk_wait local fixdt(0,16,0) =floor(12.5e6/clk_freq); stall_wait local fixdt(0,16,0) =ceil(stall_time/.04); cs_wait local fixdt(0,16,0) =ceil(cs_to_clk_edge/40); count local fixdt(0,16,0); bit_count local fixdt(0,16,0); transmit_flag local boolean; read_bit local uint16; read_temp local uint16; transmit_begin input boolean; data input fixdt(0,message_length,0); rw_bit input boolean; MISO input boolean; clk_freq constant fixdt(0,32,0) =1e6; stall_time constant fixdt(0,16,0) =4; cs_to_clk_edge constant fixdt(0,32,0) =10; message_length constant fixdt(0,16,0) =16; ready output boolean =1; READ_BIT constant boolean =1; WRITE_BIT constant boolean =0
  function ser_data = sdi_gen(word,cnt):
    | function ser_data = sdi_gen(word,cnt)
    | 
    | 
    | persistent ser_data_int;
    | if isempty(ser_data_int)
    |     ser_data_int = false;
    | end
    | 
    | 
    | if cnt == fi(1,0,5,0)
    |     ser_data_int = logical(bitget(word, 16));
    | elseif cnt == fi(2,0,5,0)
    |     ser_data_int = logical(bitget(word, 15));
    | elseif cnt == fi(3,0,5,0)
    |     ser_data_int = logical(bitget(word, 14));
    | elseif cnt == fi(4,0,5,0)
    |     ser_data_int = logical(bitget(word, 13));
    | elseif cnt == fi(5,0,5,0)
    |     ser_data_int = logical(bitget(word, 12));
    | elseif cnt == fi(6,0,5,0)
    |     ser_data_int = logical(bitget(word, 11));
    | elseif cnt == fi(7,0,5,0)
    |     ser_data_int = logical(bitget(word, 10));
    | elseif cnt == fi(8,0,5,0)
    |     ser_data_int = logical(bitget(word, 9));
    | elseif cnt == fi(9,0,5,0)
    |     ser_data_int = logical(bitget(word, 8));
    | elseif cnt == fi(10,0,5,0)
    |     ser_data_int = logical(bitget(word, 7));
    | elseif cnt == fi(11,0,5,0)
    |     ser_data_int = logical(bitget(word, 6));
    | elseif cnt == fi(12,0,5,0)
    |     ser_data_int = logical(bitget(word, 5));
    | elseif cnt == fi(13,0,5,0)
    |     ser_data_int = logical(bitget(word, 4));
    | elseif cnt == fi(14,0,5,0)
    |     ser_data_int = logical(bitget(word, 3));
    | elseif cnt == fi(15,0,5,0)
    |     ser_data_int = logical(bitget(word, 2));
    | elseif cnt == fi(16,0,5,0)
    |     ser_data_int = logical(bitget(word, 1));    
    | else
    |     ser_data_int = true;
    | end
    | 
    | ser_data = ser_data_int;
